simulink model "untitled1"  (Simulink 7.2)
settings: Solver=ode45  StartTime=0.0  StopTime=10.0  RelTol=1e-3
settings Model: Creator=Student  LastModifiedBy=Student

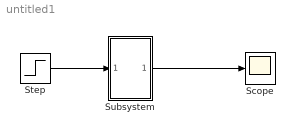
== system untitled1 ==
  Scope : Scope
      settings: TimeRange=10  YMin=0  YMax=1.5
  Step : Step  SampleTime=0
  Subsystem : Subsystem  mask{a=5}
      mask prompts: a "Parametrul a"
      mask CallbackString:
      | if str2num(get_param(gcb,'a'))<0
      |     error('Sistemul este instabil')
      | end
  wires:
  Step/1 -> Subsystem/1(In1)
  Subsystem/1(Out1) -> Scope/1

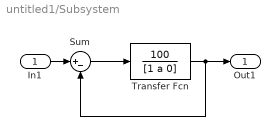
== system untitled1/Subsystem ==
  In1 : Inport  OutDataType=sfix(16)  OutScaling=2^0
  Sum : Sum  Inputs=|+-  OutDataType=sfix(16)  OutScaling=2^0
  Transfer Fcn : TransferFcn  Numerator=[100]  Denominator=[1 a 0]
  Out1 : Outport  OutDataType=sfix(16)  OutScaling=2^0
  wires:
  In1/1 -> Sum/1
  Sum/1 -> Transfer Fcn/1
  Transfer Fcn/1 -> Out1/1, Sum/2
